simulink model "genera_misure"  (R2021a)
settings: Solver=FixedStepAuto  StartTime=0.0  StopTime=10.0  FixedStep=Tc  RelTol=1e-3
values from neighbouring files (symbols this model uses):
  Tc = 0.01    [esercizio2.m]
settings Model: Creator=Giorgio  LastModifiedBy=Giorgio

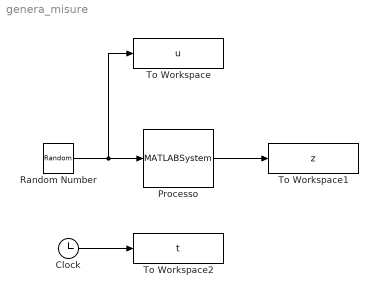
== system genera_misure ==
  Clock : Clock
  Processo : MATLABSystem  System=linSysObj  SimulateUsing=Interpreted execution
      mask Type: linSysObj
      mask Display:
      | disp('Black box');
      | port_label('input',1,'u');
      | port_label('output',1,'y');
  Random Number : RandomNumber  SampleTime=Tc
  To Workspace : ToWorkspace  VariableName=u  SampleTime=-1
      settings: Save2DSignal=2-D array (concatenate along first dimension)
  To Workspace1 : ToWorkspace  VariableName=z  SampleTime=-1
      settings: Save2DSignal=2-D array (concatenate along first dimension)
  To Workspace2 : ToWorkspace  VariableName=t  SampleTime=-1
      settings: Save2DSignal=2-D array (concatenate along first dimension)
  wires:
  Random Number/1 -> To Workspace/1, Processo/1
  Processo/1 -> To Workspace1/1
  Clock/1 -> To Workspace2/1
